simulink model "current_controller"  (R2018b)
settings: Solver=VariableStepAuto  StartTime=0.0  StopTime=10.0  RelTol=1e-3
undefined symbols (not defined in the file): Ld, Lq, Phia, Pn
settings Model: Creator=81803  LastModifiedBy=81803

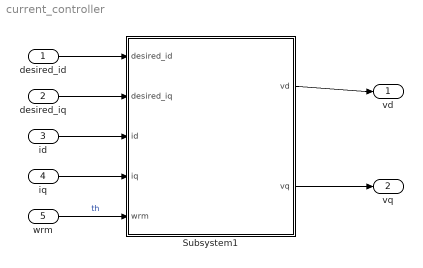
== system current_controller ==
  desired_id : Inport
  desired_iq : Inport  Port=2
  id : Inport  Port=3
  iq : Inport  Port=4
  wrm : Inport  Port=5
  Subsystem1 : Subsystem
  vd : Outport
  vq : Outport  Port=2
  wires:
  desired_id/1 -> Subsystem1/1(desired_id)
  desired_iq/1 -> Subsystem1/2(desired_iq)
  id/1 -> Subsystem1/3(id)
  iq/1 -> Subsystem1/4(iq)
  wrm/1 -> Subsystem1/5(wrm)  "th"
  Subsystem1/1(vd) -> vd/1
  Subsystem1/2(vq) -> vq/1

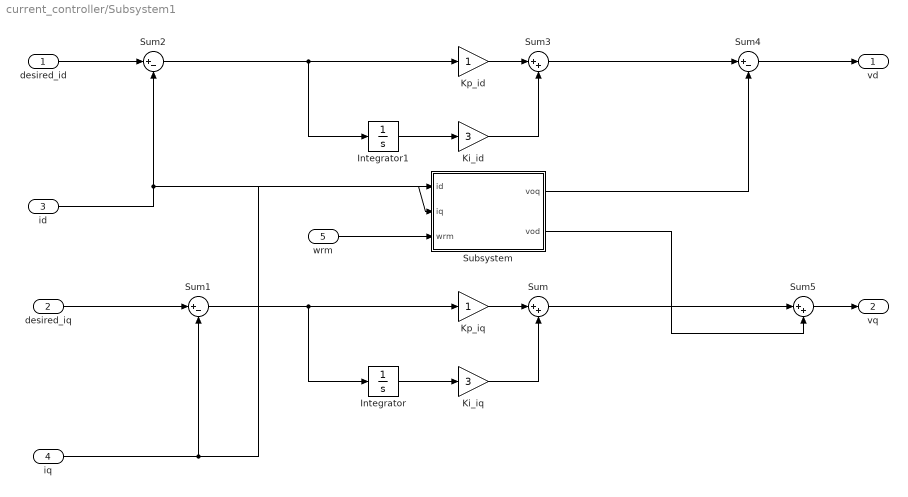
== system current_controller/Subsystem1 ==
  desired_id : Inport
  desired_iq : Inport  Port=2
  id : Inport  Port=3
  iq : Inport  Port=4
  wrm : Inport  Port=5
  Integrator : Integrator
  Integrator1 : Integrator
  Ki_id : Gain  Gain=3
  Ki_iq : Gain  Gain=3
  Kp_id : Gain
  Kp_iq : Gain
  Subsystem : Subsystem
  Sum : Sum  Inputs=|++
  Sum1 : Sum  Inputs=|+-
  Sum2 : Sum  Inputs=|+-
  Sum3 : Sum  Inputs=|++
  Sum4 : Sum  Inputs=|+-
  Sum5 : Sum  Inputs=|++
  vd : Outport
  vq : Outport  Port=2
  wires:
  Integrator/1 -> Ki_iq/1
  Sum2/1 -> Integrator1/1, Kp_id/1
  desired_iq/1 -> Sum1/1
  Subsystem/2(vod) -> Sum5/2
  desired_id/1 -> Sum2/1
  Sum3/1 -> Sum4/1
  Kp_id/1 -> Sum3/1
  Kp_iq/1 -> Sum/1
  Ki_iq/1 -> Sum/2
  iq/1 -> Subsystem/1(id), Sum1/2
  Sum1/1 -> Integrator/1, Kp_iq/1
  Integrator1/1 -> Ki_id/1
  Ki_id/1 -> Sum3/2
  id/1 -> Subsystem/2(iq), Sum2/2
  Sum/1 -> Sum5/1
  Sum4/1 -> vd/1
  Sum5/1 -> vq/1
  wrm/1 -> Subsystem/3(wrm)
  Subsystem/1(voq) -> Sum4/2

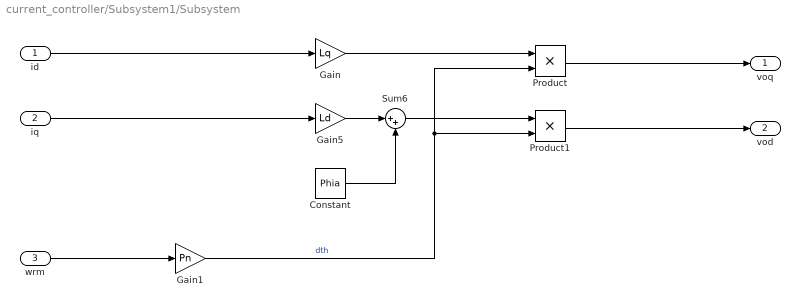
== system current_controller/Subsystem1/Subsystem ==
  id : Inport
  iq : Inport  Port=2
  wrm : Inport  Port=3
  Constant : Constant  Value=Phia
  Gain : Gain  Gain=Lq
  Gain1 : Gain  Gain=Pn
  Gain5 : Gain  Gain=Ld
  Product : Product
  Product1 : Product
  Sum6 : Sum  Inputs=|++
  voq : Outport
  vod : Outport  Port=2
  wires:
  Sum6/1 -> Product1/1
  Constant/1 -> Sum6/2
  wrm/1 -> Gain1/1
  Gain/1 -> Product/1
  Gain1/1 -> Product/2, Product1/2  "dth"
  Gain5/1 -> Sum6/1
  Product/1 -> voq/1
  iq/1 -> Gain5/1
  Product1/1 -> vod/1
  id/1 -> Gain/1
